simulink model "MLP_networks"  (Simulink 7.7)
settings: Solver=ode45  StartTime=0.0  StopTime=10.0  RelTol=1e-3
libraries: neural x1629
(part 29 of 39)

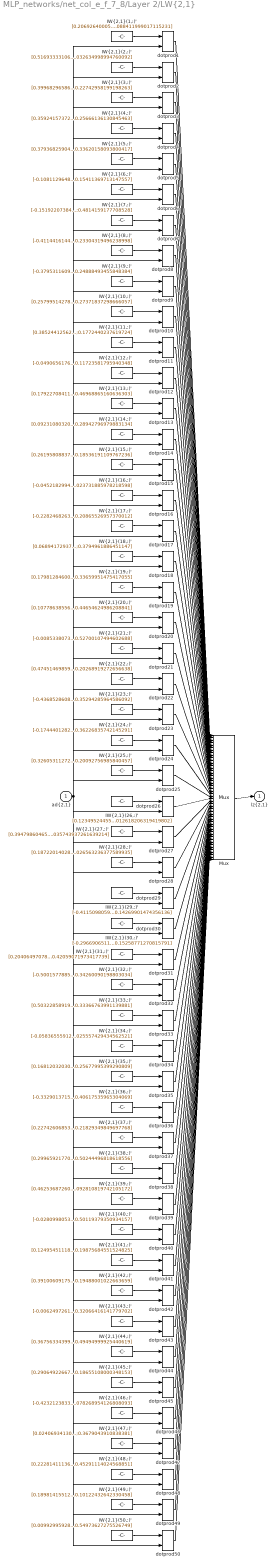
== system MLP_networks/net_col_e_f_7_8/Layer 2/LW{2,1} ==
  "ad{2,1}" : Inport  PortDimensions=30
      mask Display: e = 0.06;c1 = [120 230 180]/255;c2 = ([120 230 180]+0)/(256+128);c3 = ([120 230 180]+128)/(256+128);patch([0 1 1 0],[0 0 1 1],c1);patch([0 1 1 1-e 1-e 0+e],[0 0 1 1-e 0+e 0+e],c2);patch([0 0 1 1-e 0+e 0+e],[0 1 1 1-e 1-e 0+e],c3);plot([0 1 1 0 0],[0 0 1 1 0]);
  "IW{2,1}(1,:)'" : Constant  Value=[0.20692640005088983;-0.34878412555224553;-0.098978085881790467;0.1239813254580672;-0.041219083091532237;0.12973180000559953;0.3597297334552032;0.28955712496533176;-0.49067709101335988;0.40242056808744819;0.47396167328631478;-0.11750212984297377;-0.27318717199919562;0.37569898615283015;-0.066702934207950426;-0.082480292129323216;-0.21086887690163914;-0.40101764225037528;-0.57801263360594024;-0.047889550760827029;-0.38039231989748112;-0.037782110712844368;-0.20078431580798686;-0.18832419405514539;-0.39433313062239128;-0.14168021239809128;-0.059679202041658629;0.42551877875425254;0.4905931506693807;0.088411999017115231]
      mask Display: e = 0.06;c1 = [120 150 230]/255;c2 = ([120 150 230]+0)/383;c3 = ([120 150 230]+128)/383;patch([0 1 1 0],[0 0 1 1],c1);patch([0 1 1 1-e 1-e 0+e],[0 0 1 1-e 0+e 0+e],c2);patch([0 0 1 1-e 0+e 0+e],[0 1 1 1-e 1-e 0+e],c3);plot([0 1 1 0 0],[0 0 1 1 0]);disp('weights');
  "IW{2,1}(10,:)'" : Constant  Value=[0.25799514278352698;-0.36159512340137046;0.14778815619002283;-0.52028373171716658;-0.1369203493395777;-0.26620539272713351;0.068592800996285494;-0.45997568950494583;-0.12901952455803364;-0.17798437375480891;0.33566870049049946;0.27542264698649488;0.48197571954776264;0.046854539892267601;0.42566636563032156;-0.17172494630133636;-0.14579196006868581;-0.091305536477401208;-0.09943542522406465;-0.33697473796565269;-0.38700255880363948;-0.48659580765654686;-0.046393033040832886;-0.35383741786839012;-0.077491639714510174;-0.092211428946515531;-0.18943670675452901;0.3179965751285671;0.39142517628122458;0.27371837298666057]
      mask Display: e = 0.06;c1 = [120 150 230]/255;c2 = ([120 150 230]+0)/383;c3 = ([120 150 230]+128)/383;patch([0 1 1 0],[0 0 1 1],c1);patch([0 1 1 1-e 1-e 0+e],[0 0 1 1-e 0+e 0+e],c2);patch([0 0 1 1-e 0+e 0+e],[0 1 1 1-e 1-e 0+e],c3);plot([0 1 1 0 0],[0 0 1 1 0]);disp('weights');
  "IW{2,1}(11,:)'" : Constant  Value=[0.38524412562911514;-0.30901690922831387;-0.31420847109625327;-0.19720662173998899;-0.40155965206360417;0.20704656847487807;-0.26519350885955517;-0.43822109714691726;0.54890424824628836;-0.098609182511055382;0.17467890114154316;-0.34449359047771566;0.4101041820275132;0.41429223254550557;0.062623121083977037;0.15396951916287638;-0.148507636765874;-0.36085363535407661;0.13570994341113551;0.21827939135583097;0.16551167000423805;-0.12627672631508269;0.2279733556992275;-0.54299507544587122;0.27463612887683514;-0.0096221572986817053;0.46175085334508587;0.031717687977862376;-0.18788916679844153;0.1772440237619724]
      mask Display: e = 0.06;c1 = [120 150 230]/255;c2 = ([120 150 230]+0)/383;c3 = ([120 150 230]+128)/383;patch([0 1 1 0],[0 0 1 1],c1);patch([0 1 1 1-e 1-e 0+e],[0 0 1 1-e 0+e 0+e],c2);patch([0 0 1 1-e 0+e 0+e],[0 1 1 1-e 1-e 0+e],c3);plot([0 1 1 0 0],[0 0 1 1 0]);disp('weights');
  "IW{2,1}(12,:)'" : Constant  Value=[-0.049065617672414963;-0.39236078075580116;-0.107595269621814;-0.075243674686479634;0.27109929966677571;0.23594779000874516;0.3685300193049531;-0.092834267904196729;0.39702962224230282;-0.41245104571334146;-0.14064587847890175;0.041354855974685904;-0.11705084139366202;-0.19377500915772608;0.43812606949144661;-0.37969029490787937;-0.014011182636542592;-0.45168308974719762;-0.39233729614937007;-0.31362915540695768;0.3057113257714914;0.38307593588699401;0.06330563913773006;0.51129186785363678;-0.22376888164440981;0.1705375380698049;-0.50147816217888663;0.087168054857413954;0.28339815260172324;0.11723581795940348]
      mask Display: e = 0.06;c1 = [120 150 230]/255;c2 = ([120 150 230]+0)/383;c3 = ([120 150 230]+128)/383;patch([0 1 1 0],[0 0 1 1],c1);patch([0 1 1 1-e 1-e 0+e],[0 0 1 1-e 0+e 0+e],c2);patch([0 0 1 1-e 0+e 0+e],[0 1 1 1-e 1-e 0+e],c3);plot([0 1 1 0 0],[0 0 1 1 0]);disp('weights');
  "IW{2,1}(13,:)'" : Constant  Value=[0.17922708411449639;0.2646436394239382;0.33680430568736086;0.31174318376467214;0.031012578935646545;-0.43309949618452392;-0.048795261841146263;0.16169486520778892;-0.33928600767042605;0.15443086023430744;0.092349539379421378;-0.18514509916502808;0.42160968174402969;0.5191799710051257;-0.030840671782482149;0.13665264576730987;-0.48868680756821603;0.33903574718889046;0.075593904454067343;0.36281875816489045;-0.03322857617047132;-0.22942888275092965;-0.19808174876891538;-0.23194077766372942;0.30972048606167774;-0.18661432293069269;-0.45521167435421639;0.28472273229281747;0.2265568900477879;0.46968865160636303]
      mask Display: e = 0.06;c1 = [120 150 230]/255;c2 = ([120 150 230]+0)/383;c3 = ([120 150 230]+128)/383;patch([0 1 1 0],[0 0 1 1],c1);patch([0 1 1 1-e 1-e 0+e],[0 0 1 1-e 0+e 0+e],c2);patch([0 0 1 1-e 0+e 0+e],[0 1 1 1-e 1-e 0+e],c3);plot([0 1 1 0 0],[0 0 1 1 0]);disp('weights');
  "IW{2,1}(14,:)'" : Constant  Value=[0.092310803209110392;0.1540603383946148;-0.22036437781207244;0.50464588851016456;-0.37985383904218772;-0.20510585283963509;-0.054282421736374022;0.0026813323835861744;-0.015773412353829706;-0.15897533573499531;0.27651565557296487;-0.038791422743830531;0.32358343614728285;0.13068014805271758;0.22906225065532479;0.081037361904371427;-0.39174674224456035;0.22649658042658463;0.32985806192021289;-0.22992089507222815;0.34638320340872825;-0.39402194623309861;0.20857488663165721;-0.48319960544782253;0.17792854877353398;-0.13175522881137411;-0.52319100274113739;0.45668810052651904;-0.42680001155918523;-0.28942796979883134]
      mask Display: e = 0.06;c1 = [120 150 230]/255;c2 = ([120 150 230]+0)/383;c3 = ([120 150 230]+128)/383;patch([0 1 1 0],[0 0 1 1],c1);patch([0 1 1 1-e 1-e 0+e],[0 0 1 1-e 0+e 0+e],c2);patch([0 0 1 1-e 0+e 0+e],[0 1 1 1-e 1-e 0+e],c3);plot([0 1 1 0 0],[0 0 1 1 0]);disp('weights');
  "IW{2,1}(15,:)'" : Constant  Value=[0.26195808837474943;0.41537710963572505;0.0047837035651239704;-0.45710247449367453;0.21568163261878823;-0.089728565154573697;-0.33317111050774312;0.3459840318394542;-0.39476424754415079;-0.43635543962494877;0.44407462904230899;-0.1139031925949171;-0.25786505547132565;-0.018693644421041492;0.011692254433798387;-0.23388147431067879;-0.16248956167201384;-0.093894103953839222;-0.3538492335765982;-0.16989637026313364;0.26521472892242443;-0.34140770553942507;0.18500174642836789;-0.34517219691489953;0.15644280175318523;-0.30132310486309538;0.45161580674552421;0.43948701383597555;-0.3649160598576614;0.18536191109767236]
      mask Display: e = 0.06;c1 = [120 150 230]/255;c2 = ([120 150 230]+0)/383;c3 = ([120 150 230]+128)/383;patch([0 1 1 0],[0 0 1 1],c1);patch([0 1 1 1-e 1-e 0+e],[0 0 1 1-e 0+e 0+e],c2);patch([0 0 1 1-e 0+e 0+e],[0 1 1 1-e 1-e 0+e],c3);plot([0 1 1 0 0],[0 0 1 1 0]);disp('weights');
  "IW{2,1}(16,:)'" : Constant  Value=[-0.04521829940070312;0.035343363614029483;-0.39859581753642587;-0.53920405915138003;0.53982236630341152;-0.097695368823296033;-0.26258573828790094;0.15530384923985824;-0.015309970448159521;0.17582600463512923;-0.087535077291725077;0.34359669313102725;-0.47816641471076726;-0.010017658317955671;0.11223264474087781;-0.17200465872231638;-0.24085138316808144;0.52948219900250537;-0.35231435746854595;0.54620259388338188;0.081300467289470227;0.10574161676452101;0.3257749677635044;0.32063564329505273;-0.06664772876592602;0.21205269002082033;-0.4069295924878607;0.18733768247069998;-0.28513953366070827;0.023731885978218598]
      mask Display: e = 0.06;c1 = [120 150 230]/255;c2 = ([120 150 230]+0)/383;c3 = ([120 150 230]+128)/383;patch([0 1 1 0],[0 0 1 1],c1);patch([0 1 1 1-e 1-e 0+e],[0 0 1 1-e 0+e 0+e],c2);patch([0 0 1 1-e 0+e 0+e],[0 1 1 1-e 1-e 0+e],c3);plot([0 1 1 0 0],[0 0 1 1 0]);disp('weights');
  "IW{2,1}(17,:)'" : Constant  Value=[-0.22824682639478988;-0.34450732947400342;-0.34958761246588832;0.021381966992243984;-0.48803857902209324;0.13837112822015854;0.49430131713808462;0.16448286368241749;0.47428305751571254;-0.17697303613457299;-0.18939929393339813;0.28312252815481276;0.012180886618889022;-0.14378967891641337;-0.041631463196919002;-0.067350031048686559;-0.44528365061408798;0.40855610098806311;0.075412275630957828;0.34564721445873642;0.40591779539598161;0.1301202377986943;0.11336764905194519;-0.50715303937227463;0.35805241960071671;-0.083261880001028743;0.10598512282146536;-0.41593711285926044;-0.32411186879042964;-0.20865526957370012]
      mask Display: e = 0.06;c1 = [120 150 230]/255;c2 = ([120 150 230]+0)/383;c3 = ([120 150 230]+128)/383;patch([0 1 1 0],[0 0 1 1],c1);patch([0 1 1 1-e 1-e 0+e],[0 0 1 1-e 0+e 0+e],c2);patch([0 0 1 1-e 0+e 0+e],[0 1 1 1-e 1-e 0+e],c3);plot([0 1 1 0 0],[0 0 1 1 0]);disp('weights');
  "IW{2,1}(18,:)'" : Constant  Value=[0.068941729374186911;0.29899943147827596;0.36847548087677257;-0.067223821070221124;-0.0096997362788850093;-0.34092854432457942;0.12966057619538354;-0.30054582015316111;-0.21457640556809882;-0.13610269800234895;0.4093203343088514;0.25689292548764925;-0.46429752276052094;-0.45439265482752778;0.32013666005962982;0.19233477748155262;-0.29914921832920816;-0.34539603350512621;0.14864327892011583;0.22505599303732032;0.32800867099693531;-0.18947860561767479;0.47628634010631632;-0.3073212667960914;0.26711227444531083;0.043321923467476472;-0.48037715751554599;-0.0041820919183323318;0.080063920326655727;0.3794961886451147]
      mask Display: e = 0.06;c1 = [120 150 230]/255;c2 = ([120 150 230]+0)/383;c3 = ([120 150 230]+128)/383;patch([0 1 1 0],[0 0 1 1],c1);patch([0 1 1 1-e 1-e 0+e],[0 0 1 1-e 0+e 0+e],c2);patch([0 0 1 1-e 0+e 0+e],[0 1 1 1-e 1-e 0+e],c3);plot([0 1 1 0 0],[0 0 1 1 0]);disp('weights');
  "IW{2,1}(19,:)'" : Constant  Value=[0.17981284600754149;-0.054519984190796345;0.28358690179423746;0.39447148395809645;0.17336044771330661;-0.38302080080712619;-0.22962555670105958;0.4436835215945012;0.26675673168520181;0.0023460835877967836;-0.059253437624272716;-0.34477323835242807;-0.37307600672497987;-0.25142366950414358;-0.25362205051577441;0.4370193856984983;-0.41970940297727233;-0.38069282745402111;0.35843943307771714;0.35644498184408568;0.016162770071918842;0.32894859628271494;0.16732427161273433;-0.053067850000377954;-0.0095295853897874368;-0.38951776125685378;0.37822989703670568;0.072059092825727394;-0.25635912568919883;-0.33659951475417055]
      mask Display: e = 0.06;c1 = [120 150 230]/255;c2 = ([120 150 230]+0)/383;c3 = ([120 150 230]+128)/383;patch([0 1 1 0],[0 0 1 1],c1);patch([0 1 1 1-e 1-e 0+e],[0 0 1 1-e 0+e 0+e],c2);patch([0 0 1 1-e 0+e 0+e],[0 1 1 1-e 1-e 0+e],c3);plot([0 1 1 0 0],[0 0 1 1 0]);disp('weights');
  "IW{2,1}(2,:)'" : Constant  Value=[0.51693333106245809;-0.056647453554298462;-0.21636506475474693;0.50786371005815334;-0.46070596837765371;-0.25407578547634879;-0.05308615599121401;0.29257421870708317;-0.19488251282594049;-0.27463595063227936;0.32172489550604089;0.032886266661063979;0.32004480174259642;-0.15608448532173827;0.2694114759871617;0.029461174709978773;0.15575173305668702;0.1247925703478376;0.089487032773308897;-0.35131850057060787;-0.052402872749339455;0.4030539260696126;0.50398982579100904;0.33660732197972709;-0.1305111491174028;-0.1990091376120805;-0.30307854260723649;0.46460416874279736;0.33979416670688517;0.032634998994760092]
      mask Display: e = 0.06;c1 = [120 150 230]/255;c2 = ([120 150 230]+0)/383;c3 = ([120 150 230]+128)/383;patch([0 1 1 0],[0 0 1 1],c1);patch([0 1 1 1-e 1-e 0+e],[0 0 1 1-e 0+e 0+e],c2);patch([0 0 1 1-e 0+e 0+e],[0 1 1 1-e 1-e 0+e],c3);plot([0 1 1 0 0],[0 0 1 1 0]);disp('weights');
  "IW{2,1}(20,:)'" : Constant  Value=[0.10778638556560378;0.18688000010375783;-0.11960607214083416;0.23649578976096244;-0.22523596517114505;-0.066607317767425567;-0.30051088233806816;0.1782255510912043;-0.36195950119738057;0.3321550829040783;0.11966461622171229;0.30564806158964525;-0.18195589533565168;-0.18449705979245717;-0.0041665039088435128;-0.034293246476064618;0.25948766179212512;-0.45933542063762717;-0.22043228588875979;0.47208661353081666;0.29490913062966378;0.37621464530571314;-0.13585759481080076;-0.44332501808384372;0.13685921769221612;-0.47507000781526748;0.48460444113143403;-0.43781462641886948;0.069978439067215653;0.44654624986208841]
      mask Display: e = 0.06;c1 = [120 150 230]/255;c2 = ([120 150 230]+0)/383;c3 = ([120 150 230]+128)/383;patch([0 1 1 0],[0 0 1 1],c1);patch([0 1 1 1-e 1-e 0+e],[0 0 1 1-e 0+e 0+e],c2);patch([0 0 1 1-e 0+e 0+e],[0 1 1 1-e 1-e 0+e],c3);plot([0 1 1 0 0],[0 0 1 1 0]);disp('weights');
  "IW{2,1}(21,:)'" : Constant  Value=[-0.0085338073034539105;-0.21534439801113364;-0.42791477694049368;-0.13604014801977432;-0.446513004116254;-0.13181947680025599;0.37518086255339372;-0.29323521697094951;0.32856960518279804;-0.054396911731497057;-0.23860964761308509;0.04034263369441056;-0.073771286329046115;-0.048065056797906208;-0.31074313638055773;0.30178431460370414;-0.13895414976777515;-0.46077862899343541;-0.014736807141923446;-0.36448904433364959;0.040784086522330933;0.18841170180339936;-0.027070582978472268;0.45258302416294915;-0.38655050869528396;0.38228805597861576;-0.246582686497714;0.45421328209687173;0.22392843851787506;0.52700107494602688]
      mask Display: e = 0.06;c1 = [120 150 230]/255;c2 = ([120 150 230]+0)/383;c3 = ([120 150 230]+128)/383;patch([0 1 1 0],[0 0 1 1],c1);patch([0 1 1 1-e 1-e 0+e],[0 0 1 1-e 0+e 0+e],c2);patch([0 0 1 1-e 0+e 0+e],[0 1 1 1-e 1-e 0+e],c3);plot([0 1 1 0 0],[0 0 1 1 0]);disp('weights');
  "IW{2,1}(22,:)'" : Constant  Value=[0.47451469859006079;0.10997231423457665;-0.4865796221666342;0.37020870218255569;0.19181891401085999;-0.36554166956266637;0.20442097608557569;0.054402575798912868;0.019239951804784043;-0.018067281936818003;0.36065951753192327;-0.13126008272903547;-0.062909887940032438;-0.30689234684728894;-0.093701258451697231;-0.011299727038715571;-0.36095649532169177;0.48416662042363656;-0.42087156121394376;0.036820682035746746;-0.10597347470125471;0.0089322960385902501;-0.356826615699879;-0.36791255918083815;-0.37541828477143785;-0.46782101762169809;-0.017237297884314787;0.52901956127434957;-0.034304189450448254;-0.20268919272656638]
      mask Display: e = 0.06;c1 = [120 150 230]/255;c2 = ([120 150 230]+0)/383;c3 = ([120 150 230]+128)/383;patch([0 1 1 0],[0 0 1 1],c1);patch([0 1 1 1-e 1-e 0+e],[0 0 1 1-e 0+e 0+e],c2);patch([0 0 1 1-e 0+e 0+e],[0 1 1 1-e 1-e 0+e],c3);plot([0 1 1 0 0],[0 0 1 1 0]);disp('weights');
  "IW{2,1}(23,:)'" : Constant  Value=[-0.43685286088142361;-0.07046033329475769;0.26359707151232298;0.36537086812114489;-0.43238760681781635;0.13862021026366841;-0.077526663077627442;0.26834814698489301;-0.25273473314405037;0.47134826085376863;0.11557985990187815;0.37133685072357148;0.31373647964802226;-0.42583484687332601;-0.30976249576987341;-0.24454961201289926;0.32612654693296983;-0.011094946358309441;-0.15188854906101087;0.13206622300739784;0.29101882270824592;0.2594624061612929;-0.068429654818553967;0.47808223512111486;0.27918145648279369;0.43332333863705147;0.13212955182801117;-0.034734010641744681;-0.21529557637469987;0.35294285964586092]
      mask Display: e = 0.06;c1 = [120 150 230]/255;c2 = ([120 150 230]+0)/383;c3 = ([120 150 230]+128)/383;patch([0 1 1 0],[0 0 1 1],c1);patch([0 1 1 1-e 1-e 0+e],[0 0 1 1-e 0+e 0+e],c2);patch([0 0 1 1-e 0+e 0+e],[0 1 1 1-e 1-e 0+e],c3);plot([0 1 1 0 0],[0 0 1 1 0]);disp('weights');
  "IW{2,1}(24,:)'" : Constant  Value=[-0.17444012823365548;-0.11310709220902772;0.14874804870035149;-0.031887761632281186;0.26810666508993491;0.3805172086151512;0.35705782272468961;0.134309445304094;-0.31683068663921082;0.10591216023481181;0.20390791632412225;-0.18850327641002279;0.46699268441316372;0.32043773197234321;-0.22271418026768991;0.32681502863389028;-0.23130170886293946;-0.54937959334378794;0.44987812092259716;-0.28342527032103315;0.48519760179433741;0.083160649660007344;-0.033962169480701548;0.04389454759749694;-0.064169817181577882;0.070277824564589142;-0.38812693128954745;0.24937610292243489;-0.40372827730198063;-0.36226835742145291]
      mask Display: e = 0.06;c1 = [120 150 230]/255;c2 = ([120 150 230]+0)/383;c3 = ([120 150 230]+128)/383;patch([0 1 1 0],[0 0 1 1],c1);patch([0 1 1 1-e 1-e 0+e],[0 0 1 1-e 0+e 0+e],c2);patch([0 0 1 1-e 0+e 0+e],[0 1 1 1-e 1-e 0+e],c3);plot([0 1 1 0 0],[0 0 1 1 0]);disp('weights');
  "IW{2,1}(25,:)'" : Constant  Value=[0.3260531127206806;-0.34638802451403328;-0.12059705256642995;-0.052420515550794071;0.25704821925064952;0.29528199465172356;0.002787877374711408;-0.023920009189642363;-0.36633627788249118;0.40529913049681804;0.26591749825234262;-0.33316017930868325;0.41251062576027647;0.38392397674340295;0.39380089114970679;0.2532512683411105;0.289354255389213;-0.42852708598217876;0.33383332561085494;-0.29899988755215579;-0.061261575053359087;-0.072146796086322823;0.31829890263702582;0.24593632218040354;0.051381781398100006;-0.37733058832712651;-0.405223724043414;-0.25787732957520221;0.26867479400665317;-0.20092756985840457]
      mask Display: e = 0.06;c1 = [120 150 230]/255;c2 = ([120 150 230]+0)/383;c3 = ([120 150 230]+128)/383;patch([0 1 1 0],[0 0 1 1],c1);patch([0 1 1 1-e 1-e 0+e],[0 0 1 1-e 0+e 0+e],c2);patch([0 0 1 1-e 0+e 0+e],[0 1 1 1-e 1-e 0+e],c3);plot([0 1 1 0 0],[0 0 1 1 0]);disp('weights');
  "IW{2,1}(26,:)'" : Constant  Value=[0.12349524455517442;-0.080057956141856054;-0.41096899702996881;-0.32834479398977695;-0.17054489412656468;0.15851975669455484;0.049022457668018236;0.41415922382997339;-0.34777929072109615;0.46771211446801253;0.48341752925524739;0.10314724551060821;-0.20451291295866106;0.16616696313971477;-0.054178079601731891;0.031242563746234693;-0.15745343507690593;-0.44137487714660439;-0.25738906551700574;0.40151144517664361;-0.20168503081547304;-0.47274409842345189;-0.1576806926926905;-0.25815621177346304;-0.25985431032338319;0.16341473954303398;0.30551869272483156;-0.42582523684230511;-0.41182863743324344;-0.0012618206319419802]
      mask Display: e = 0.06;c1 = [120 150 230]/255;c2 = ([120 150 230]+0)/383;c3 = ([120 150 230]+128)/383;patch([0 1 1 0],[0 0 1 1],c1);patch([0 1 1 1-e 1-e 0+e],[0 0 1 1-e 0+e 0+e],c2);patch([0 0 1 1-e 0+e 0+e],[0 1 1 1-e 1-e 0+e],c3);plot([0 1 1 0 0],[0 0 1 1 0]);disp('weights');
  "IW{2,1}(27,:)'" : Constant  Value=[0.39479860465220185;0.091541846855625553;0.21608302522427567;0.33433073695514975;-0.15169529017772013;0.078749011451528822;0.03144410496081676;0.26305501084569716;0.40486779092014924;-0.44657533453591208;-0.35496999578532451;-0.10129312430179273;0.21243307659091498;0.3177627541538729;-0.2542677188985874;-0.063343731936092149;0.19500087027396668;0.30332347277110866;-0.30786178844846612;-0.37124216410551514;-0.20417755100300972;0.44433231646768623;0.36575567943120718;-0.56845855021750746;0.26029245742076229;0.10531509901387424;0.13752146408280969;0.12755544051923295;-0.48860599745644462;-0.035743937261639214]
      mask Display: e = 0.06;c1 = [120 150 230]/255;c2 = ([120 150 230]+0)/383;c3 = ([120 150 230]+128)/383;patch([0 1 1 0],[0 0 1 1],c1);patch([0 1 1 1-e 1-e 0+e],[0 0 1 1-e 0+e 0+e],c2);patch([0 0 1 1-e 0+e 0+e],[0 1 1 1-e 1-e 0+e],c3);plot([0 1 1 0 0],[0 0 1 1 0]);disp('weights');
  "IW{2,1}(28,:)'" : Constant  Value=[0.18722014028883882;-0.38746170133976776;0.18975523358005134;-0.39604618852856321;-0.39055703717358875;0.46353373894531502;0.14890294389263495;0.16075106535746941;-0.23427660958156274;0.48141991603583073;-0.36864729116691464;0.35590367037646137;-0.16956059456557726;0.24333250489197855;-0.05963612520617563;0.40973003014175235;-0.15612992366837264;-0.36432733852066523;0.34841655624149898;0.41649791832445104;-0.18850427214670143;0.2846263407691636;-0.25005067965304584;-0.11598538784199663;0.050239192501436908;-0.026260084713605535;0.3969782617612686;0.40367752802383988;-0.075886370750741144;0.026563236377589935]
      mask Display: e = 0.06;c1 = [120 150 230]/255;c2 = ([120 150 230]+0)/383;c3 = ([120 150 230]+128)/383;patch([0 1 1 0],[0 0 1 1],c1);patch([0 1 1 1-e 1-e 0+e],[0 0 1 1-e 0+e 0+e],c2);patch([0 0 1 1-e 0+e 0+e],[0 1 1 1-e 1-e 0+e],c3);plot([0 1 1 0 0],[0 0 1 1 0]);disp('weights');
  "IW{2,1}(29,:)'" : Constant  Value=[-0.41150980593819858;-0.49900981707901809;0.044667929894832273;-0.28627294802574005;-0.11358876001710091;-0.39610782529961625;0.14095969174004161;0.011320142196528209;0.48484174959859117;-0.29961128479911647;0.21770477505594985;0.13113864859265212;-0.022763305470973796;-0.058282565617675842;-0.22811278191709775;0.40214481869417279;-0.23146847757061484;-0.50979539875975033;-0.22412468580117784;0.047799458856465339;-0.10275439914559822;-0.55896210445110106;0.25138237573347222;0.12285395428622706;-0.50907942371430503;0.48367689135912811;0.044711328534607485;0.10932853125834509;0.086813915219554283;-0.14269901474356136]
      mask Display: e = 0.06;c1 = [120 150 230]/255;c2 = ([120 150 230]+0)/383;c3 = ([120 150 230]+128)/383;patch([0 1 1 0],[0 0 1 1],c1);patch([0 1 1 1-e 1-e 0+e],[0 0 1 1-e 0+e 0+e],c2);patch([0 0 1 1-e 0+e 0+e],[0 1 1 1-e 1-e 0+e],c3);plot([0 1 1 0 0],[0 0 1 1 0]);disp('weights');
  "IW{2,1}(3,:)'" : Constant  Value=[0.39968296586131252;-0.26949477983792292;-0.36280819068437697;-0.28030637824029703;-0.2740054492401614;0.18655463897020433;0.26547834092333611;-0.22418366309693233;-0.26512965361945079;-0.40030826846009476;-0.040111644791402459;-0.10481531565431945;-0.20013140144678368;-0.38841932919253475;0.11093564865823929;0.43766347433649594;0.043532641151452438;0.31597897514081996;-0.098235178110639559;0.082006720858306389;0.41151032598087367;-0.17943811705841684;0.44169918642283218;0.40566573755001045;-0.37397564933983668;-0.37047432260404456;0.39484986833887425;-0.12478606023984265;-0.15211490360027694;0.22742958199198263]
      mask Display: e = 0.06;c1 = [120 150 230]/255;c2 = ([120 150 230]+0)/383;c3 = ([120 150 230]+128)/383;patch([0 1 1 0],[0 0 1 1],c1);patch([0 1 1 1-e 1-e 0+e],[0 0 1 1-e 0+e 0+e],c2);patch([0 0 1 1-e 0+e 0+e],[0 1 1 1-e 1-e 0+e],c3);plot([0 1 1 0 0],[0 0 1 1 0]);disp('weights');
  "IW{2,1}(30,:)'" : Constant  Value=[-0.2966906511552504;0.11747130970964373;-0.49124595731774767;-0.21259654448093751;-0.13285467627852643;-0.045888174914016359;0.31418016516729846;-0.36905638623041942;0.28734697023523476;0.37411583016445932;-0.35862135488773222;0.30493490548384061;0.42148237090716567;-0.42812668479077504;0.21506888104364053;-0.1496511298771328;0.33517369394323859;-0.4922569513503039;-0.23117932769302132;0.4253049390174295;-0.36413310798494208;-0.061563322797895163;-0.083758438864501225;0.054278236709449493;0.28369742475566045;0.04611294033255104;0.077964648813593898;0.051887612977833591;0.41806202927733865;-0.15258771270815791]
      mask Display: e = 0.06;c1 = [120 150 230]/255;c2 = ([120 150 230]+0)/383;c3 = ([120 150 230]+128)/383;patch([0 1 1 0],[0 0 1 1],c1);patch([0 1 1 1-e 1-e 0+e],[0 0 1 1-e 0+e 0+e],c2);patch([0 0 1 1-e 0+e 0+e],[0 1 1 1-e 1-e 0+e],c3);plot([0 1 1 0 0],[0 0 1 1 0]);disp('weights');
  "IW{2,1}(31,:)'" : Constant  Value=[0.20406497078524968;-0.43611805540038057;-0.23605220252870651;-0.37422793864075904;-0.27018346281873273;0.4610470810126604;-0.34175657368329926;-0.026235615552713434;0.36994659113679207;-0.32803370579551838;-0.17997098516368176;-0.26268495022253235;0.066639865428010966;0.16808978907277755;0.17889901235976133;-0.16852147314648072;-0.16910470057157273;0.057598343633531127;0.3244920099526164;0.45348633334306299;0.31603693985595255;-0.34420158495111425;-0.4714596613131562;-0.10555140418280448;-0.085292022478128088;0.19944982382705859;0.17532501853387902;-0.47296045395187547;-0.011823546985776125;0.42059071973417739]
      mask Display: e = 0.06;c1 = [120 150 230]/255;c2 = ([120 150 230]+0)/383;c3 = ([120 150 230]+128)/383;patch([0 1 1 0],[0 0 1 1],c1);patch([0 1 1 1-e 1-e 0+e],[0 0 1 1-e 0+e 0+e],c2);patch([0 0 1 1-e 0+e 0+e],[0 1 1 1-e 1-e 0+e],c3);plot([0 1 1 0 0],[0 0 1 1 0]);disp('weights');
  "IW{2,1}(32,:)'" : Constant  Value=[-0.50015778851815174;0.1834331298651265;0.30359486340719094;0.10982562690850475;0.005379045100671046;0.49496428746294108;0.47618119072996917;-0.049515974500581483;0.42714857334426654;-0.19452318270119501;0.37125565443096104;0.022937442799857242;-0.31909172521945744;0.14242614915488419;0.47885555834057114;-0.28615454420129677;0.0098098819236362815;-0.41845019178596421;0.3145954511682868;-0.15393165156593183;0.29362110224107035;-0.085994524125396141;-0.090455611740342223;-0.49518906058459089;-0.31173185817619908;-0.24567968453684511;0.095564398141187168;0.11202858390013397;-0.23494225327855411;0.34260090198803034]
      mask Display: e = 0.06;c1 = [120 150 230]/255;c2 = ([120 150 230]+0)/383;c3 = ([120 150 230]+128)/383;patch([0 1 1 0],[0 0 1 1],c1);patch([0 1 1 1-e 1-e 0+e],[0 0 1 1-e 0+e 0+e],c2);patch([0 0 1 1-e 0+e 0+e],[0 1 1 1-e 1-e 0+e],c3);plot([0 1 1 0 0],[0 0 1 1 0]);disp('weights');
  "IW{2,1}(33,:)'" : Constant  Value=[0.50322858919625491;0.11278877793590854;-0.043909866620707894;-0.040246151396034442;0.2226341986123731;0.16269269719560936;-0.05256643629023626;-0.43560474049364389;0.3249163270805121;0.14016971542025805;-0.091679746112435317;-0.39628968473753357;-0.37108520761653685;-0.18791785837857175;-0.22835785415595283;0.048197143472726689;-0.19894974869912885;0.34456931663313589;-0.28905628464090843;-0.28313398646529769;-0.35910631748226679;-0.45833005370838464;-0.37091374077049266;0.17536078884018563;-0.51010288123161251;0.16498692269749685;0.50092795593123007;0.050304739627509726;-0.069276288578979051;0.33366763991139881]
      mask Display: e = 0.06;c1 = [120 150 230]/255;c2 = ([120 150 230]+0)/383;c3 = ([120 150 230]+128)/383;patch([0 1 1 0],[0 0 1 1],c1);patch([0 1 1 1-e 1-e 0+e],[0 0 1 1-e 0+e 0+e],c2);patch([0 0 1 1-e 0+e 0+e],[0 1 1 1-e 1-e 0+e],c3);plot([0 1 1 0 0],[0 0 1 1 0]);disp('weights');
  "IW{2,1}(34,:)'" : Constant  Value=[-0.058365559124964585;-0.343269059684361;0.23691859702493975;-0.23890078995137032;-0.075847939573769105;-0.35287818751785743;0.11306300051425532;-0.44178295546087309;0.30602867649819698;0.45849167086965681;-0.3965211378074523;-0.24546627014691494;0.12761144536331542;-0.27074105952463445;-0.072522943953271815;-0.12342819427194127;0.055571916104978636;0.37285602953557495;0.28555055487692277;0.35510290092907454;0.39658814825747102;-0.46225394401910758;0.37829484698308402;0.25416718760823886;-0.40205892416354688;0.47998316092240867;-0.0014110736744630179;-0.32303758704028479;-0.045349234049867841;0.0025557429434562521]
      mask Display: e = 0.06;c1 = [120 150 230]/255;c2 = ([120 150 230]+0)/383;c3 = ([120 150 230]+128)/383;patch([0 1 1 0],[0 0 1 1],c1);patch([0 1 1 1-e 1-e 0+e],[0 0 1 1-e 0+e 0+e],c2);patch([0 0 1 1-e 0+e 0+e],[0 1 1 1-e 1-e 0+e],c3);plot([0 1 1 0 0],[0 0 1 1 0]);disp('weights');
  "IW{2,1}(35,:)'" : Constant  Value=[0.16812032030970026;0.11222429401170071;0.24232437961834458;0.27545651539447225;0.25926684974168063;0.0084245805473293373;-0.31508811635622447;-0.0025096628733374962;0.30613982439909188;0.29695174965911109;0.055949063561341661;-0.44944256580568021;-0.31831938126763704;0.32039217296089378;0.25197054403718921;-0.30440261011807546;0.46526499817924977;-0.18153726029996911;0.47862421316581988;0.00073781911591174734;-0.31928640119456692;0.19396533946211686;-0.31024991533130403;0.39656031819788945;0.32142751331189073;-0.065239457450802937;-0.44567868546834699;0.003150060508631816;-0.50662816380018294;-0.25677995399290809]
      mask Display: e = 0.06;c1 = [120 150 230]/255;c2 = ([120 150 230]+0)/383;c3 = ([120 150 230]+128)/383;patch([0 1 1 0],[0 0 1 1],c1);patch([0 1 1 1-e 1-e 0+e],[0 0 1 1-e 0+e 0+e],c2);patch([0 0 1 1-e 0+e 0+e],[0 1 1 1-e 1-e 0+e],c3);plot([0 1 1 0 0],[0 0 1 1 0]);disp('weights');
  "IW{2,1}(36,:)'" : Constant  Value=[-0.33290137157743716;-0.3821088661609362;-0.21490190396083095;-0.34979608974120147;0.39562937521026342;0.071810910502952782;0.27973016450362165;0.065084085130221236;0.192202338971246;-0.18420097673420532;-0.44177417193445423;-0.32143315363367725;-0.12545474052768935;-0.10405844841465983;0.056075998831222072;-0.19543007908416682;-0.15046205422253778;-0.40621840454575409;0.42776936995786052;0.26100357594807033;-0.32716048065317282;0.41625163368487483;-0.40788738075569658;-0.36056026471918545;-0.10205767988050078;0.067335740912969649;0.16710415439277532;0.40136677349519095;0.22747080778064141;0.40617535965304069]
      mask Display: e = 0.06;c1 = [120 150 230]/255;c2 = ([120 150 230]+0)/383;c3 = ([120 150 230]+128)/383;patch([0 1 1 0],[0 0 1 1],c1);patch([0 1 1 1-e 1-e 0+e],[0 0 1 1-e 0+e 0+e],c2);patch([0 0 1 1-e 0+e 0+e],[0 1 1 1-e 1-e 0+e],c3);plot([0 1 1 0 0],[0 0 1 1 0]);disp('weights');
  "IW{2,1}(37,:)'" : Constant  Value=[0.22742606853119923;0.05363091783030699;0.26661046902908792;-0.079502990615816949;0.26402682915057374;0.21500181633412566;0.49685925462443564;0.10849973396334717;0.42381663222001509;0.41445745108725884;0.14844170373357421;-0.48205562821039533;-0.25181867681983611;0.05524815977741418;-0.32552409644466146;-0.41773934940277629;-0.19982427677735126;0.24820622696978875;-0.27832357152279885;-0.2608108242851927;-0.47901942955033266;-0.43756260534782065;-0.32448053884219025;-0.37488073252537557;0.23432803176480246;-0.059724828053824133;0.1127518986780371;-0.077936730614158164;0.38016199549376928;-0.21829349849697768]
      mask Display: e = 0.06;c1 = [120 150 230]/255;c2 = ([120 150 230]+0)/383;c3 = ([120 150 230]+128)/383;patch([0 1 1 0],[0 0 1 1],c1);patch([0 1 1 1-e 1-e 0+e],[0 0 1 1-e 0+e 0+e],c2);patch([0 0 1 1-e 0+e 0+e],[0 1 1 1-e 1-e 0+e],c3);plot([0 1 1 0 0],[0 0 1 1 0]);disp('weights');
  "IW{2,1}(38,:)'" : Constant  Value=[0.29965921770000564;-0.084819758360605749;0.25120792786045304;0.086165089606520376;0.02015204987799965;0.19609832146372017;-0.43059819463937038;0.35072862647285696;-0.097021925135886825;0.38048643780852431;0.38296164039261116;0.28480430054817657;0.10782560106608213;0.31840743173266933;0.30336869745206901;0.24304238648125734;-0.24575655994617837;0.20066482369760358;-0.48013929308856051;0.001674108714817134;-0.29368740074975608;0.17238295364075421;0.052446146387182549;0.18748202215641158;0.22572014228336265;-0.4576731874148755;0.49758794038697701;-0.40219479023934085;0.051985902914823474;0.50244496818618556]
      mask Display: e = 0.06;c1 = [120 150 230]/255;c2 = ([120 150 230]+0)/383;c3 = ([120 150 230]+128)/383;patch([0 1 1 0],[0 0 1 1],c1);patch([0 1 1 1-e 1-e 0+e],[0 0 1 1-e 0+e 0+e],c2);patch([0 0 1 1-e 0+e 0+e],[0 1 1 1-e 1-e 0+e],c3);plot([0 1 1 0 0],[0 0 1 1 0]);disp('weights');
  "IW{2,1}(39,:)'" : Constant  Value=[0.46253687260756388;0.29515951750532476;0.329370458298479;-0.054627743809303658;-0.13007275209818553;0.1261472424633443;0.10394136040717597;0.17816626733923474;-0.20263655339336281;0.14774731087869036;0.50929386147099664;0.35360207119324411;0.19901678825235128;0.23071782170448063;0.28585946146276531;-0.43668702614973492;0.105889913922238;-0.43948609041166942;0.46363828756843745;0.26209627903136418;0.39090724731062704;0.12986443567739561;0.38412335799415043;0.2538879861835513;0.18683331538494785;-0.38507742934145045;0.41133801530096892;0.22695923580442545;-0.14822888683102647;-0.092810819742105172]
      mask Display: e = 0.06;c1 = [120 150 230]/255;c2 = ([120 150 230]+0)/383;c3 = ([120 150 230]+128)/383;patch([0 1 1 0],[0 0 1 1],c1);patch([0 1 1 1-e 1-e 0+e],[0 0 1 1-e 0+e 0+e],c2);patch([0 0 1 1-e 0+e 0+e],[0 1 1 1-e 1-e 0+e],c3);plot([0 1 1 0 0],[0 0 1 1 0]);disp('weights');
  "IW{2,1}(4,:)'" : Constant  Value=[0.35924157372045928;0.06459506006057858;-0.084590279631242021;0.20587734624419973;-0.0097524276671683442;0.2526974799947157;-0.12006409992235786;0.013278385173005348;-0.25574215900063518;-0.44755255835724989;0.082028130526621515;0.54768309800040171;-0.3246051477601804;-0.47062925427458563;0.014239107299711432;-0.19624214094802356;0.42107887207075423;-0.37730057778083059;-0.04984410653418244;0.4103473442170632;-0.30950134514804956;-0.20536048716514854;-0.17133357287383932;-0.062347459182039856;-0.34428299681985974;0.32343317599977151;-0.39672094656778306;0.47551445004923287;-0.041017108588179189;-0.25666136130845463]
      mask Display: e = 0.06;c1 = [120 150 230]/255;c2 = ([120 150 230]+0)/383;c3 = ([120 150 230]+128)/383;patch([0 1 1 0],[0 0 1 1],c1);patch([0 1 1 1-e 1-e 0+e],[0 0 1 1-e 0+e 0+e],c2);patch([0 0 1 1-e 0+e 0+e],[0 1 1 1-e 1-e 0+e],c3);plot([0 1 1 0 0],[0 0 1 1 0]);disp('weights');
  "IW{2,1}(40,:)'" : Constant  Value=[-0.028099805302707323;-0.29201159902195611;-0.30379020716669519;0.13029308450003754;0.27206545547252697;-0.0043094687334352391;0.36082955469478406;-0.29938935269965022;0.12887633759628345;-0.10751199717419888;-0.0036234117856460391;0.40355501424736451;0.28750270021144081;0.27284211145486803;0.023268841691787282;0.40780329254097086;-0.39281297906432738;-0.17361606630860249;-0.49432770258871606;0.2489325084886396;-0.063205138818003145;0.4658292830452988;0.41417318084451021;-0.32731682675596724;0.37298760152094496;0.10422114665437655;0.20814235183867613;-0.11936068761010125;-0.2738929602000274;-0.50119379350934157]
      mask Display: e = 0.06;c1 = [120 150 230]/255;c2 = ([120 150 230]+0)/383;c3 = ([120 150 230]+128)/383;patch([0 1 1 0],[0 0 1 1],c1);patch([0 1 1 1-e 1-e 0+e],[0 0 1 1-e 0+e 0+e],c2);patch([0 0 1 1-e 0+e 0+e],[0 1 1 1-e 1-e 0+e],c3);plot([0 1 1 0 0],[0 0 1 1 0]);disp('weights');
  "IW{2,1}(41,:)'" : Constant  Value=[0.12495451118948644;-0.469746304541726;0.44222792691957952;0.38365323238428756;-0.12613148910139696;0.38176416097966592;0.067031425658773958;-0.078381000998299172;-0.20887602464773164;-0.067885036378594277;-0.36969981728748014;-0.060965196152132285;-0.34827952037861276;-0.013878381548895785;-0.17097989530736299;0.42755057611931824;0.29611542777153732;0.51912177669086168;0.15680911990980229;0.40688442426305393;-0.46325050657844352;0.091360981776117997;0.31972184426970912;0.19475878067638205;0.093625170149642639;0.46440585330286438;-0.011513735684631427;0.32516066813830569;0.13329011278719108;-0.19875684551524825]
      mask Display: e = 0.06;c1 = [120 150 230]/255;c2 = ([120 150 230]+0)/383;c3 = ([120 150 230]+128)/383;patch([0 1 1 0],[0 0 1 1],c1);patch([0 1 1 1-e 1-e 0+e],[0 0 1 1-e 0+e 0+e],c2);patch([0 0 1 1-e 0+e 0+e],[0 1 1 1-e 1-e 0+e],c3);plot([0 1 1 0 0],[0 0 1 1 0]);disp('weights');
  "IW{2,1}(42,:)'" : Constant  Value=[0.39100609175431694;0.4551880054865054;-0.27956913810344536;-0.13725232958658523;0.31732717286387518;-0.25934980957595205;-0.2628172153796603;0.068169116645129854;-0.27675339077254879;0.33337116091515889;-0.0123868994889604;-0.3483645684258741;0.35884879206940823;0.30129232588975974;-0.18978921478317742;-0.067989654103865746;-0.43514302729391935;0.4516594051956061;0.31345779637478599;-0.076304776759774151;0.4362913704496611;0.31083888737748355;-0.43232162747315839;-0.19080835916367367;-0.052230962050476573;-0.33743009413042191;0.047298004365901404;0.24288642251401796;-0.048849722582875024;-0.19488001022663659]
      mask Display: e = 0.06;c1 = [120 150 230]/255;c2 = ([120 150 230]+0)/383;c3 = ([120 150 230]+128)/383;patch([0 1 1 0],[0 0 1 1],c1);patch([0 1 1 1-e 1-e 0+e],[0 0 1 1-e 0+e 0+e],c2);patch([0 0 1 1-e 0+e 0+e],[0 1 1 1-e 1-e 0+e],c3);plot([0 1 1 0 0],[0 0 1 1 0]);disp('weights');
  "IW{2,1}(43,:)'" : Constant  Value=[-0.0062497261759218792;-0.40587362955107198;0.12791260779108313;0.41179039880084178;0.51561157894503418;-0.37099783630321431;-0.22880843998250128;-0.20111081068423386;0.19726398900245343;0.21842339733112276;-0.2689905882477418;-0.42023859693092336;-0.099581922120293292;0.27683446366798353;-0.032666519974203771;-0.23706306592355583;-0.13997531834981766;0.083450500885925108;-0.31750081196403224;0.2139312799414039;-0.46304576109555562;0.16021816446520723;-0.14985989098193905;-0.42441144473140707;-0.32234318992904071;0.15741056218528046;-0.40056780140081477;-0.37539269547132359;-0.049613557702175452;0.32066416141779702]
      mask Display: e = 0.06;c1 = [120 150 230]/255;c2 = ([120 150 230]+0)/383;c3 = ([120 150 230]+128)/383;patch([0 1 1 0],[0 0 1 1],c1);patch([0 1 1 1-e 1-e 0+e],[0 0 1 1-e 0+e 0+e],c2);patch([0 0 1 1-e 0+e 0+e],[0 1 1 1-e 1-e 0+e],c3);plot([0 1 1 0 0],[0 0 1 1 0]);disp('weights');
  "IW{2,1}(44,:)'" : Constant  Value=[0.36756334399376461;-0.33051553715596915;-0.17849436137715738;0.3983822192547084;0.29352696651625826;0.025582607531849603;0.19778925907356051;0.14431622191312193;-0.21798321990400393;-0.15724683764571107;0.39195100320442594;-0.40879005680024633;-0.090495508259857083;0.07824746104268579;0.4144670028145902;0.097246461146126215;0.4966789461181223;0.29148943435550939;-0.23980168354578088;0.33346295697822148;-0.189205493360696;0.12082136064774682;-0.13952274719113847;-0.31145998702708499;0.46996154514332383;0.20641885534169202;0.30771322175317312;0.23744005128515633;0.26972839681675759;0.49494999925440619]
      mask Display: e = 0.06;c1 = [120 150 230]/255;c2 = ([120 150 230]+0)/383;c3 = ([120 150 230]+128)/383;patch([0 1 1 0],[0 0 1 1],c1);patch([0 1 1 1-e 1-e 0+e],[0 0 1 1-e 0+e 0+e],c2);patch([0 0 1 1-e 0+e 0+e],[0 1 1 1-e 1-e 0+e],c3);plot([0 1 1 0 0],[0 0 1 1 0]);disp('weights');
  "IW{2,1}(45,:)'" : Constant  Value=[0.29064922667046056;-0.10487358403942601;-0.3939953403152805;-0.49872603340165661;0.25979971178965111;-0.18835046914663836;0.50744363305479068;-0.33252796727971412;0.38071907584270154;0.11926417574899195;0.15786739517321219;-0.31694285836737424;-0.25755331485453575;0.3316788372736954;-0.21550443637794653;-0.23190478390592226;0.51244392447722575;0.10092522196960209;-0.4184371042497505;0.045224045890953309;-0.45578451646468815;-0.020590129725874953;0.049691594233803468;0.085721963562902764;0.43519207110630365;-0.1349321915076519;-0.041951670819811923;0.31228138245734993;0.13675955768343309;-0.18655108000348153]
      mask Display: e = 0.06;c1 = [120 150 230]/255;c2 = ([120 150 230]+0)/383;c3 = ([120 150 230]+128)/383;patch([0 1 1 0],[0 0 1 1],c1);patch([0 1 1 1-e 1-e 0+e],[0 0 1 1-e 0+e 0+e],c2);patch([0 0 1 1-e 0+e 0+e],[0 1 1 1-e 1-e 0+e],c3);plot([0 1 1 0 0],[0 0 1 1 0]);disp('weights');
  "IW{2,1}(46,:)'" : Constant  Value=[-0.42321238336572647;-0.30158545620997751;0.38102688892100439;0.20938475473759469;0.3146239381059982;-0.29008606481527666;0.20019421325625633;0.49409147416561705;0.010360654976385461;0.34704896296753934;-0.017945354672448365;0.27427500003267385;-0.25797796189908029;0.359400240411128;-0.25368725026338218;-0.17644992010561927;0.42735686439566228;0.1640138193866883;-0.22566678402672583;-0.19402666504260524;0.27186170967650874;0.40599150226682568;-0.27244713181457719;0.35770532213568146;-0.26354258225708055;-0.45873935435352398;0.12677422596170604;-0.044694693097860047;0.24732441860201484;-0.078268954126808093]
      mask Display: e = 0.06;c1 = [120 150 230]/255;c2 = ([120 150 230]+0)/383;c3 = ([120 150 230]+128)/383;patch([0 1 1 0],[0 0 1 1],c1);patch([0 1 1 1-e 1-e 0+e],[0 0 1 1-e 0+e 0+e],c2);patch([0 0 1 1-e 0+e 0+e],[0 1 1 1-e 1-e 0+e],c3);plot([0 1 1 0 0],[0 0 1 1 0]);disp('weights');
  "IW{2,1}(47,:)'" : Constant  Value=[0.024069341302313446;0.029197842234870156;0.11779845205567188;0.25069705699013339;0.37310328188115877;-0.099571875301879553;0.16534406518598399;-0.16853543046692537;-0.062530790235435008;-0.20928841469177936;-0.25495897353177299;-0.043604373960521921;0.19017960376715207;0.35852778200941104;0.45446013330388552;-0.13748250277543617;-0.47339792237809358;-0.18204371443966955;0.31144150010430288;-0.22028513405902544;-0.44829561370607401;0.4416757868427002;-0.38365937556816565;0.24068188196439907;-0.46346475843283547;0.023574087042326268;0.49991921147647594;-0.012477068787406178;0.17627736513338127;0.3679043910838381]
      mask Display: e = 0.06;c1 = [120 150 230]/255;c2 = ([120 150 230]+0)/383;c3 = ([120 150 230]+128)/383;patch([0 1 1 0],[0 0 1 1],c1);patch([0 1 1 1-e 1-e 0+e],[0 0 1 1-e 0+e 0+e],c2);patch([0 0 1 1-e 0+e 0+e],[0 1 1 1-e 1-e 0+e],c3);plot([0 1 1 0 0],[0 0 1 1 0]);disp('weights');
  "IW{2,1}(48,:)'" : Constant  Value=[0.22281411136206195;0.025942434874401191;0.054399550614745239;0.035574484902397195;0.46675054606451893;-0.43300910454394631;-0.11335796062734931;0.38056703507748757;0.1318986878638973;0.37238571930892617;0.041044663912616547;-0.21867134457895318;-0.386576214780042;-0.29274525944186341;-0.12603402852655649;0.071795169935409436;0.4323969900696687;-0.39845243443884165;-0.29502133124262364;-0.27746155885517931;-0.43982854892324602;0.26257406860633437;0.3125248636262109;0.30983613010407718;0.16154366013800953;0.20752608393426394;-0.32657493253834435;-0.33588547363396354;0.19975562936254301;0.45291114024568851]
      mask Display: e = 0.06;c1 = [120 150 230]/255;c2 = ([120 150 230]+0)/383;c3 = ([120 150 230]+128)/383;patch([0 1 1 0],[0 0 1 1],c1);patch([0 1 1 1-e 1-e 0+e],[0 0 1 1-e 0+e 0+e],c2);patch([0 0 1 1-e 0+e 0+e],[0 1 1 1-e 1-e 0+e],c3);plot([0 1 1 0 0],[0 0 1 1 0]);disp('weights');
  "IW{2,1}(49,:)'" : Constant  Value=[0.18981415512183866;0.0089311124388671403;-0.29502721105554697;0.50826735621510177;0.50456148868518336;0.20213681384675852;0.14670602835171223;-0.012442596487875147;0.08336981793304396;-0.19908883639356756;0.27832293861681828;-0.38673437613159783;-0.036053405982465606;-0.20274019021124845;0.34132023753857255;-0.42016915945318489;-0.2320317918418624;-0.11089494826396516;0.11270075526003109;-0.38476632939498923;-0.24715363976880692;-0.30868100464601178;0.13137982799593662;0.4663603279477741;0.50856662374095607;-0.08295021351078867;0.42139938957353351;0.37282530667012775;0.34419728079893303;0.10122432642330458]
      mask Display: e = 0.06;c1 = [120 150 230]/255;c2 = ([120 150 230]+0)/383;c3 = ([120 150 230]+128)/383;patch([0 1 1 0],[0 0 1 1],c1);patch([0 1 1 1-e 1-e 0+e],[0 0 1 1-e 0+e 0+e],c2);patch([0 0 1 1-e 0+e 0+e],[0 1 1 1-e 1-e 0+e],c3);plot([0 1 1 0 0],[0 0 1 1 0]);disp('weights');
  "IW{2,1}(5,:)'" : Constant  Value=[0.37936825904296945;0.23289430693347291;0.045446768082242711;-0.35034498138820375;-0.35762110700803024;-0.04540332518930984;-0.41890112132559926;0.41361918405071252;-0.010536665183002364;0.30369596507513713;-0.41519469108058404;0.35196176032782633;0.25880860410648049;0.35195268395885254;0.34991963792860648;0.075972946198644614;-0.41204850386923902;-0.12481235123775603;0.043499600889344049;-0.37032309239959693;-0.13081735989999874;-0.038783549792050447;-0.016058137919528457;0.06939418983386611;-0.2981115550237563;0.30074950090826308;0.40428101835552271;-0.27873928742168469;0.41379392808458981;0.33620158093800417]
      mask Display: e = 0.06;c1 = [120 150 230]/255;c2 = ([120 150 230]+0)/383;c3 = ([120 150 230]+128)/383;patch([0 1 1 0],[0 0 1 1],c1);patch([0 1 1 1-e 1-e 0+e],[0 0 1 1-e 0+e 0+e],c2);patch([0 0 1 1-e 0+e 0+e],[0 1 1 1-e 1-e 0+e],c3);plot([0 1 1 0 0],[0 0 1 1 0]);disp('weights');
  "IW{2,1}(50,:)'" : Constant  Value=[0.0099299592897046964;0.061501690199812317;0.29872773629086735;-0.12788072781345705;0.21820741069511945;-0.10485838355011358;-0.16099724613426791;0.14031024822061902;0.43836727714066936;0.095189521618169751;0.35887964575755571;0.30541943568304902;-0.025226408809458669;0.37832191093937834;0.57593788798745726;0.25078576112716794;0.48786220277704595;0.12097548879274506;-0.1270427584364226;-0.083494027177491159;-0.20316577289562088;-0.521638070971009;-0.041104779658754705;-0.029815910841284987;0.11116221524572044;-0.34040637170044613;0.028762333990475546;0.45221745487035803;-0.34648800584797429;0.54973627275526749]
      mask Display: e = 0.06;c1 = [120 150 230]/255;c2 = ([120 150 230]+0)/383;c3 = ([120 150 230]+128)/383;patch([0 1 1 0],[0 0 1 1],c1);patch([0 1 1 1-e 1-e 0+e],[0 0 1 1-e 0+e 0+e],c2);patch([0 0 1 1-e 0+e 0+e],[0 1 1 1-e 1-e 0+e],c3);plot([0 1 1 0 0],[0 0 1 1 0]);disp('weights');
  "IW{2,1}(6,:)'" : Constant  Value=[-0.10811296489528031;-0.018279494630695746;-0.04283061529541346;-0.44924165682995754;0.38607503549068389;0.11933393751163485;0.33166253395289264;0.30567422356621105;0.35415256849165622;-0.33633313531878045;0.1621862227874997;-0.21501446279772377;-0.36154628075981932;-0.35715218357277634;-0.19087079087679082;-0.27967432227415151;-0.40283049908641244;0.049373960836611448;-0.45764272813928136;0.15675294845630625;-0.042838185915685861;0.15728458835992573;-0.42526205340669221;0.26466138257083432;-0.35566919014447762;-0.14279870531287384;0.39620616502753214;0.35126819765121808;-0.36960965808619151;0.15411369713147557]
      mask Display: e = 0.06;c1 = [120 150 230]/255;c2 = ([120 150 230]+0)/383;c3 = ([120 150 230]+128)/383;patch([0 1 1 0],[0 0 1 1],c1);patch([0 1 1 1-e 1-e 0+e],[0 0 1 1-e 0+e 0+e],c2);patch([0 0 1 1-e 0+e 0+e],[0 1 1 1-e 1-e 0+e],c3);plot([0 1 1 0 0],[0 0 1 1 0]);disp('weights');
  "IW{2,1}(7,:)'" : Constant  Value=[-0.15192207384025957;-0.19025536976326596;0.031880353062139849;0.058548453087543625;-0.10426794223781079;-0.022748923959271521;0.048118509105105754;-0.17876362300434667;-0.15636888358535272;0.50466917202338357;-0.51878504512850643;0.1744099385332645;-0.29989981513744807;-0.44377819004266206;-0.084601154803407061;-0.082284218733614897;0.14560664328373793;0.0032897907927425529;-0.46921467526571209;-0.37373304347046304;-0.40003540525199005;0.20741281908862924;0.026017114510083993;0.40895448424621644;0.38655420068864521;0.37462129763913388;-0.10195950076977787;0.44945940154126407;0.34985351557583694;0.4814159177708528]
      mask Display: e = 0.06;c1 = [120 150 230]/255;c2 = ([120 150 230]+0)/383;c3 = ([120 150 230]+128)/383;patch([0 1 1 0],[0 0 1 1],c1);patch([0 1 1 1-e 1-e 0+e],[0 0 1 1-e 0+e 0+e],c2);patch([0 0 1 1-e 0+e 0+e],[0 1 1 1-e 1-e 0+e],c3);plot([0 1 1 0 0],[0 0 1 1 0]);disp('weights');
  "IW{2,1}(8,:)'" : Constant  Value=[-0.41144161442801436;0.29238286162764132;-0.36777164258589295;-0.0057490173029810443;0.32591330100236121;-0.32016166223286296;-0.26537994541952559;-0.38104751458823072;0.12125539393537779;0.072197188619828365;0.17486230563259983;-0.37984861900956718;0.31039283746498042;-0.10452798410508894;-0.12221601342274403;0.096951213895968447;-0.17538195443478963;-0.079411614544730405;0.25446171988145416;0.4641227311006953;0.19155375327936933;0.18769113702780851;-0.27348708788430404;0.35414486030318471;0.52854138730650801;0.19357069774879299;-0.40714985948129606;0.14178501377881075;0.40985815335887787;0.23304319496238998]
      mask Display: e = 0.06;c1 = [120 150 230]/255;c2 = ([120 150 230]+0)/383;c3 = ([120 150 230]+128)/383;patch([0 1 1 0],[0 0 1 1],c1);patch([0 1 1 1-e 1-e 0+e],[0 0 1 1-e 0+e 0+e],c2);patch([0 0 1 1-e 0+e 0+e],[0 1 1 1-e 1-e 0+e],c3);plot([0 1 1 0 0],[0 0 1 1 0]);disp('weights');
  "IW{2,1}(9,:)'" : Constant  Value=[-0.3795311609524985;0.21623417015464594;-0.21374144104204368;0.45983093386441609;-0.041248530338517518;0.21733046122851832;-0.13571947230739226;0.24880113689260572;0.10422653301859768;-0.46165790736045748;0.11022694629669515;-0.31081219332309507;-0.4161212373227236;-0.39075235128504543;-0.55287904856316306;-0.41259149305681991;-0.12013115986791892;-0.37762568318719802;-0.22314974470045326;0.3986206530656487;0.25591437141368278;-0.30278177382821714;0.19768149867158777;-0.25184211114039445;0.065359345188550994;0.12103662317016309;-0.00089065526161710934;-0.2671148265762916;-0.22721168363952954;-0.24888493455848384]
      mask Display: e = 0.06;c1 = [120 150 230]/255;c2 = ([120 150 230]+0)/383;c3 = ([120 150 230]+128)/383;patch([0 1 1 0],[0 0 1 1],c1);patch([0 1 1 1-e 1-e 0+e],[0 0 1 1-e 0+e 0+e],c2);patch([0 0 1 1-e 0+e 0+e],[0 1 1 1-e 1-e 0+e],c3);plot([0 1 1 0 0],[0 0 1 1 0]);disp('weights');
  Mux : Mux  Inputs=50
      mask Display: e = 0.06;c1 = [120 150 230]/255;c2 = ([120 150 230]+0)/383;c3 = ([120 150 230]+128)/383;patch([0 1 1 0],[0 0 1 1],c1);patch([0 1 1 1-e 1-e 0+e],[0 0 1 1-e 0+e 0+e],c2);patch([0 0 1 1-e 0+e 0+e],[0 1 1 1-e 1-e 0+e],c3);plot([0 1 1 0 0],[0 0 1 1 0]);disp('Mux');
  dotprod{1..50} (50 alike) : neural/Weight Functions/dotprod  SystemSampleTime=-1
  "lz{2,1}" : Outport
      mask Display: e = 0.06;c1 = [120 230 180]/255;c2 = ([120 230 180]+0)/(256+128);c3 = ([120 230 180]+128)/(256+128);patch([0 1 1 0],[0 0 1 1],c1);patch([0 1 1 1-e 1-e 0+e],[0 0 1 1-e 0+e 0+e],c2);patch([0 0 1 1-e 0+e 0+e],[0 1 1 1-e 1-e 0+e],c3);plot([0 1 1 0 0],[0 0 1 1 0]);
  wires:
  "IW{2,1}(1,:)'"/1 -> dotprod1/1
  "ad{2,1}"/1 -> dotprod1/2, dotprod2/2, dotprod3/2, dotprod4/2, dotprod5/2, dotprod6/2, dotprod7/2, dotprod8/2, dotprod9/2, dotprod10/2, dotprod11/2, dotprod12/2, dotprod13/2, dotprod14/2, dotprod15/2, dotprod16/2, dotprod17/2, dotprod18/2, dotprod19/2, dotprod20/2, dotprod21/2, dotprod22/2, dotprod23/2, dotprod24/2, dotprod25/2, dotprod26/2, dotprod27/2, dotprod28/2, dotprod29/2, dotprod30/2, dotprod31/2, dotprod32/2, dotprod33/2, dotprod34/2, dotprod35/2, dotprod36/2, dotprod37/2, dotprod38/2, dotprod39/2, dotprod40/2, dotprod41/2, dotprod42/2, dotprod43/2, dotprod44/2, dotprod45/2, dotprod46/2, dotprod47/2, dotprod48/2, dotprod49/2, dotprod50/2
  dotprod1/1 -> Mux/1
  "IW{2,1}(2,:)'"/1 -> dotprod2/1
  dotprod2/1 -> Mux/2
  "IW{2,1}(3,:)'"/1 -> dotprod3/1
  dotprod3/1 -> Mux/3
  "IW{2,1}(4,:)'"/1 -> dotprod4/1
  dotprod4/1 -> Mux/4
  "IW{2,1}(5,:)'"/1 -> dotprod5/1
  dotprod5/1 -> Mux/5
  "IW{2,1}(6,:)'"/1 -> dotprod6/1
  dotprod6/1 -> Mux/6
  "IW{2,1}(7,:)'"/1 -> dotprod7/1
  dotprod7/1 -> Mux/7
  "IW{2,1}(8,:)'"/1 -> dotprod8/1
  dotprod8/1 -> Mux/8
  "IW{2,1}(9,:)'"/1 -> dotprod9/1
  dotprod9/1 -> Mux/9
  "IW{2,1}(10,:)'"/1 -> dotprod10/1
  dotprod10/1 -> Mux/10
  "IW{2,1}(11,:)'"/1 -> dotprod11/1
  dotprod11/1 -> Mux/11
  "IW{2,1}(12,:)'"/1 -> dotprod12/1
  dotprod12/1 -> Mux/12
  "IW{2,1}(13,:)'"/1 -> dotprod13/1
  dotprod13/1 -> Mux/13
  "IW{2,1}(14,:)'"/1 -> dotprod14/1
  dotprod14/1 -> Mux/14
  "IW{2,1}(15,:)'"/1 -> dotprod15/1
  dotprod15/1 -> Mux/15
  "IW{2,1}(16,:)'"/1 -> dotprod16/1
  dotprod16/1 -> Mux/16
  "IW{2,1}(17,:)'"/1 -> dotprod17/1
  dotprod17/1 -> Mux/17
  "IW{2,1}(18,:)'"/1 -> dotprod18/1
  dotprod18/1 -> Mux/18
  "IW{2,1}(19,:)'"/1 -> dotprod19/1
  dotprod19/1 -> Mux/19
  "IW{2,1}(20,:)'"/1 -> dotprod20/1
  dotprod20/1 -> Mux/20
  "IW{2,1}(21,:)'"/1 -> dotprod21/1
  dotprod21/1 -> Mux/21
  "IW{2,1}(22,:)'"/1 -> dotprod22/1
  dotprod22/1 -> Mux/22
  "IW{2,1}(23,:)'"/1 -> dotprod23/1
  dotprod23/1 -> Mux/23
  "IW{2,1}(24,:)'"/1 -> dotprod24/1
  dotprod24/1 -> Mux/24
  "IW{2,1}(25,:)'"/1 -> dotprod25/1
  dotprod25/1 -> Mux/25
  "IW{2,1}(26,:)'"/1 -> dotprod26/1
  dotprod26/1 -> Mux/26
  "IW{2,1}(27,:)'"/1 -> dotprod27/1
  dotprod27/1 -> Mux/27
  "IW{2,1}(28,:)'"/1 -> dotprod28/1
  dotprod28/1 -> Mux/28
  "IW{2,1}(29,:)'"/1 -> dotprod29/1
  dotprod29/1 -> Mux/29
  "IW{2,1}(30,:)'"/1 -> dotprod30/1
  dotprod30/1 -> Mux/30
  "IW{2,1}(31,:)'"/1 -> dotprod31/1
  dotprod31/1 -> Mux/31
  "IW{2,1}(32,:)'"/1 -> dotprod32/1
  dotprod32/1 -> Mux/32
  "IW{2,1}(33,:)'"/1 -> dotprod33/1
  dotprod33/1 -> Mux/33
  "IW{2,1}(34,:)'"/1 -> dotprod34/1
  dotprod34/1 -> Mux/34
  "IW{2,1}(35,:)'"/1 -> dotprod35/1
  dotprod35/1 -> Mux/35
  "IW{2,1}(36,:)'"/1 -> dotprod36/1
  dotprod36/1 -> Mux/36
  "IW{2,1}(37,:)'"/1 -> dotprod37/1
  dotprod37/1 -> Mux/37
  "IW{2,1}(38,:)'"/1 -> dotprod38/1
  dotprod38/1 -> Mux/38
  "IW{2,1}(39,:)'"/1 -> dotprod39/1
  dotprod39/1 -> Mux/39
  "IW{2,1}(40,:)'"/1 -> dotprod40/1
  dotprod40/1 -> Mux/40
  "IW{2,1}(41,:)'"/1 -> dotprod41/1
  dotprod41/1 -> Mux/41
  "IW{2,1}(42,:)'"/1 -> dotprod42/1
  dotprod42/1 -> Mux/42
  "IW{2,1}(43,:)'"/1 -> dotprod43/1
  dotprod43/1 -> Mux/43
  "IW{2,1}(44,:)'"/1 -> dotprod44/1
  dotprod44/1 -> Mux/44
  "IW{2,1}(45,:)'"/1 -> dotprod45/1
  dotprod45/1 -> Mux/45
  "IW{2,1}(46,:)'"/1 -> dotprod46/1
  dotprod46/1 -> Mux/46
  "IW{2,1}(47,:)'"/1 -> dotprod47/1
  dotprod47/1 -> Mux/47
  "IW{2,1}(48,:)'"/1 -> dotprod48/1
  dotprod48/1 -> Mux/48
  "IW{2,1}(49,:)'"/1 -> dotprod49/1
  dotprod49/1 -> Mux/49
  "IW{2,1}(50,:)'"/1 -> dotprod50/1
  dotprod50/1 -> Mux/50
  Mux/1 -> "lz{2,1}"/1
